simulink model "ADAPTIVEpidLYP"  (R2018b)
settings: Solver=ode3  StartTime=0.0  StopTime=2000  FixedStep=.01  RelTol=1e-3  EnableMultiTasking=on
StopFcn:
  | figure();
  | subplot(2,1,1)
  | plot(out.time , out.signals.values(:,1:2)) ;
  | xlabel('Time') ;
  | ylabel('Amp');
  | title('Adaptive PID based on lyponove');
  | grid on
  | legend('Ym','Y');
  | 
  | subplot(2,1,2)
  | plot(out.time , out.signals.values(:,3)) ;
  | xlabel('Time') ;
  | ylabel('Amp');
  | title('Adaptive PID based on lyponove - effort conrtol');
  | grid on
  | legend('U');
  | 
  | figure();
  | plot(parametersPID.time , parametersPID.signals.values ) ;
  | xlabel('Time') ;
  | ylabel('Amp');
  | title('Adaptive PID based on lyponove - parameters convergence');
  | grid on
  | legend('F','Q1','Q2');
settings Model: Creator=FaraDars  LastModifiedBy=Arash
settings DataIOCC: LimitDataPoints=on  SaveFormat=Array
settings OptimizationCC: LifeSpan=inf
settings DebuggingCC: SFUnexpectedBacktrackingDiag=warning  SFNoUnconditionalDefaultTransitionDiag=warning  SFExecutionAtInitializationDiag=none
settings HardwareCC: ProdBitPerPointer=32  ProdBitPerSizeT=32  ProdBitPerPtrDiffT=32  ProdLargestAtomicFloat=None  ProdIntDivRoundTo=Undefined  ProdEndianess=Unspecified  ProdWordSize=32  ProdHWDeviceType=32-bit Generic
settings ModelReferenceCC: PropagateSignalLabelsOutOfModel=off
settings SFSimCC: SimUseLocalCustomCode=off
settings RTWCC: RTWUseLocalCustomCode=off
settings CodeAppCC: StateflowObjectComments=on
settings GRTTargetCC: TargetLangStandard=C89/C90 (ANSI)  GeneratePreprocessorConditionals=Disable all
settings ConfigComp: CovMetricSettings=dw  CovHtmlReporting=on  CovSaveCumulativeToWorkspaceVar=on  CovSaveSingleToWorkspaceVar=on  CovExternalEMLEnable=off

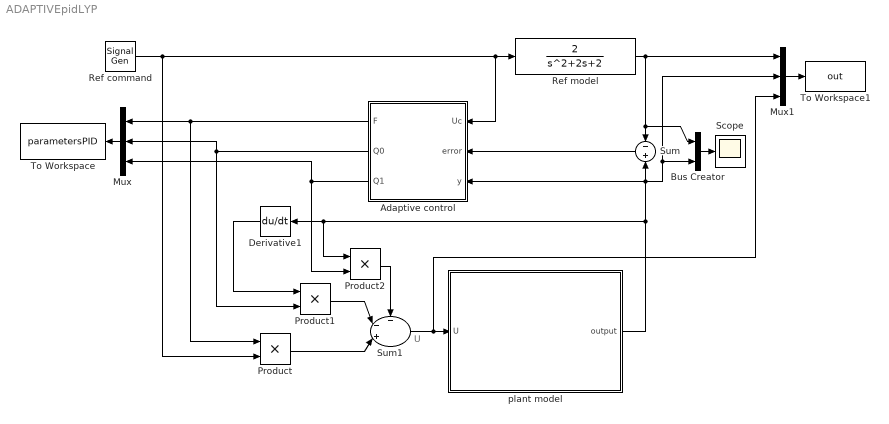
== system ADAPTIVEpidLYP ==
  note: U
  Adaptive control : Subsystem
  Bus Creator : BusCreator  Inputs=2
  Derivative1 : Derivative
  Mux : Mux  Inputs=3
  Mux1 : Mux  Inputs=3
  Product : Product
  Product1 : Product
  Product2 : Product
  "Ref command " : SignalGenerator  WaveForm=square  Frequency=.01/2
  Ref model : TransferFcn  Numerator=[2]  Denominator=[1 2 2]
  Scope : Scope
  Sum : Sum  Inputs=-|+
  Sum1 : Sum  Inputs=--+|
  To Workspace : ToWorkspace  VariableName=parametersPID  SaveFormat=Structure With Time  SampleTime=-1
  To Workspace1 : ToWorkspace  VariableName=out  SaveFormat=Structure With Time  SampleTime=-1
  plant model : Subsystem
  wires:
  "Ref command "/1 -> Ref model/1, Adaptive control/1(Uc), Product/2
  Ref model/1 -> Mux1/1, Bus Creator/1, Sum/1
  Sum1/1 -> Mux1/3, plant model/1(U)
  Product/1 -> Sum1/3
  Product1/1 -> Sum1/2
  Adaptive control/2(Q0) -> Product1/2, Mux/2
  Derivative1/1 -> Product1/1
  Product2/1 -> Sum1/1
  Sum/1 -> Adaptive control/2(" error")
  plant model/1(output) -> Mux1/2, Bus Creator/2, Adaptive control/3(y), Sum/2, Product2/1, Derivative1/1
  Adaptive control/1(F) -> Mux/1, Product/1
  Adaptive control/3(Q1) -> Product2/2, Mux/3
  Bus Creator/1 -> Scope/1
  Mux/1 -> To Workspace/1
  Mux1/1 -> To Workspace1/1

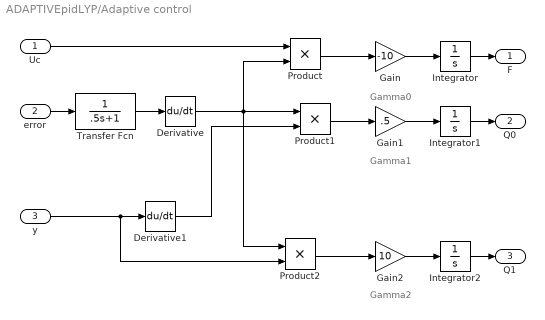
== system ADAPTIVEpidLYP/Adaptive control ==
  note: Gamma2
  note: Gamma1
  note: Gamma0
  Uc : Inport
  " error" : Inport  Port=2
  y : Inport  Port=3
  Derivative : Derivative
  Derivative1 : Derivative
  Gain : Gain  Gain=-10
  Gain1 : Gain  Gain=.5
  Gain2 : Gain  Gain=10
  Integrator : Integrator
  Integrator1 : Integrator
  Integrator2 : Integrator
  Product : Product
  Product1 : Product
  Product2 : Product
  Transfer Fcn : TransferFcn  Denominator=[.5 1]
  F : Outport
  Q0 : Outport  Port=2
  Q1 : Outport  Port=3
  wires:
  Integrator/1 -> F/1
  Integrator2/1 -> Q1/1
  Integrator1/1 -> Q0/1
  Uc/1 -> Product/1
  Derivative/1 -> Product2/1, Product1/1, Product/2
  Product2/1 -> Gain2/1
  Gain2/1 -> Integrator2/1
  Gain1/1 -> Integrator1/1
  Product1/1 -> Gain1/1
  Gain/1 -> Integrator/1
  Product/1 -> Gain/1
  y/1 -> Product2/2, Derivative1/1
  Derivative1/1 -> Product1/2
  " error"/1 -> Transfer Fcn/1
  Transfer Fcn/1 -> Derivative/1

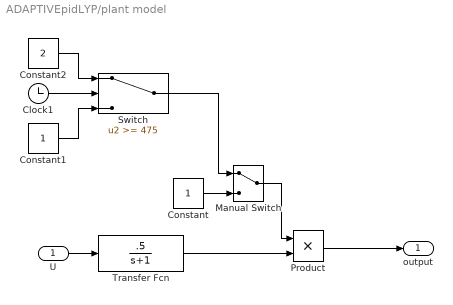
== system ADAPTIVEpidLYP/plant model ==
  U : Inport
  Clock1 : Clock
  Constant : Constant
  Constant1 : Constant
  Constant2 : Constant  Value=2
  Manual Switch : ManualSwitch
  Product : Product
  Switch : Switch  Threshold=475
  Transfer Fcn : TransferFcn  Numerator=[.5]  Denominator=[1 1]
  output : Outport
  wires:
  Manual Switch/1 -> Product/1
  Constant/1 -> Manual Switch/2
  Switch/1 -> Manual Switch/1
  Constant1/1 -> Switch/3
  Constant2/1 -> Switch/1
  Clock1/1 -> Switch/2
  Product/1 -> output/1
  Transfer Fcn/1 -> Product/2
  U/1 -> Transfer Fcn/1
